simulink model "CAE_FPslx"  (R2023b)
settings: Solver=VariableStepAuto  StartTime=0.0  StopTime=10.0  MaxStep=0.001  RelTol=1e-3
settings Model: Creator=Wojciech Zub  LastModifiedBy=Wojciech Zub

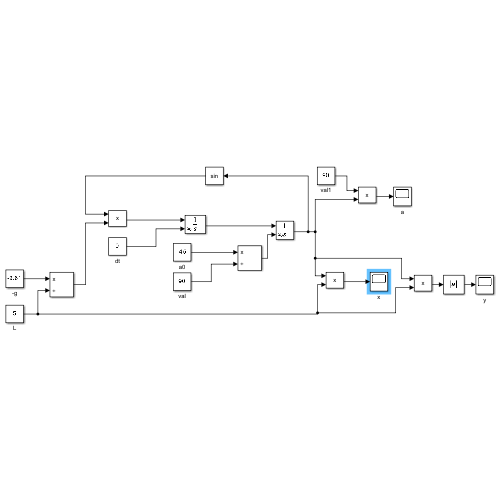
[thumbnail: Simulink's stored preview of the top-level diagram]
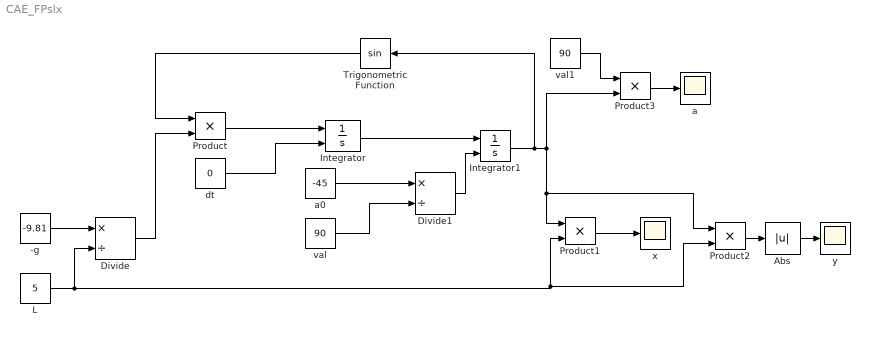
== system CAE_FPslx ==
  -g : Constant  Value=-9.81
  Abs : Abs  SaturateOnIntegerOverflow=off
  Divide : Product  Inputs=*/
  Divide1 : Product  Inputs=*/
  Integrator : Integrator  InitialConditionSource=external
  Integrator1 : Integrator  InitialConditionSource=external
  L : Constant  Value=5
  Product{,1..3} (4 alike) : Product
  Trigonometric Function : Trigonometry
  a : Scope
  a0 : Constant  Value=-45
  dt : Constant  Value=0
  val : Constant  Value=90
  val1 : Constant  Value=90
  x : Scope
  y : Scope
  wires:
  Integrator/1 -> Integrator1/1
  Trigonometric Function/1 -> Product/1
  dt/1 -> Integrator/2
  Divide1/1 -> Integrator1/2
  Divide/1 -> Product/2
  -g/1 -> Divide/1
  L/1 -> Product1/2, Product2/2, Divide/2
  Product/1 -> Integrator/1
  Product1/1 -> x/1
  Integrator1/1 -> Trigonometric Function/1, Product3/2, Product1/1, Product2/1
  Product2/1 -> Abs/1
  val/1 -> Divide1/2
  a0/1 -> Divide1/1
  val1/1 -> Product3/1
  Product3/1 -> a/1
  Abs/1 -> y/1
